simulink model "computed_torque_rl"  (R2021b)
settings: Solver=VariableStepAuto  StartTime=0  StopTime=3.6  RelTol=1e-3
values from neighbouring files (symbols this model uses):
  kd = 2*sqrt(kp)    [model_using.m]
  kp = 50700    [model_using.m]
  n = 100    [model_using.m]
libraries: slpidlib x4
settings Model: SimulationMode=accelerator  Creator=dell  LastModifiedBy=Admin
settings DataIOCC: SaveFormat=StructureWithTime
settings OptimizationCC: BlockReduction=off  BufferReuse=off
settings DebuggingCC: AlgebraicLoopMsg=none  UnconnectedInputMsg=none  UnconnectedOutputMsg=none  UnconnectedLineMsg=none
settings ExplorerConfigSet: SimMechanicsOpenEditorOnUpdate=off

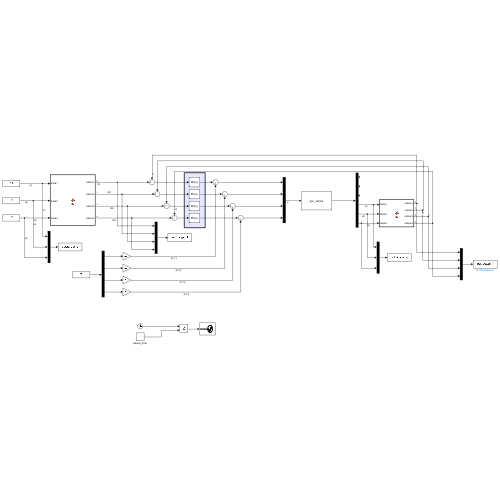
[thumbnail: Simulink's stored preview of the top-level diagram]
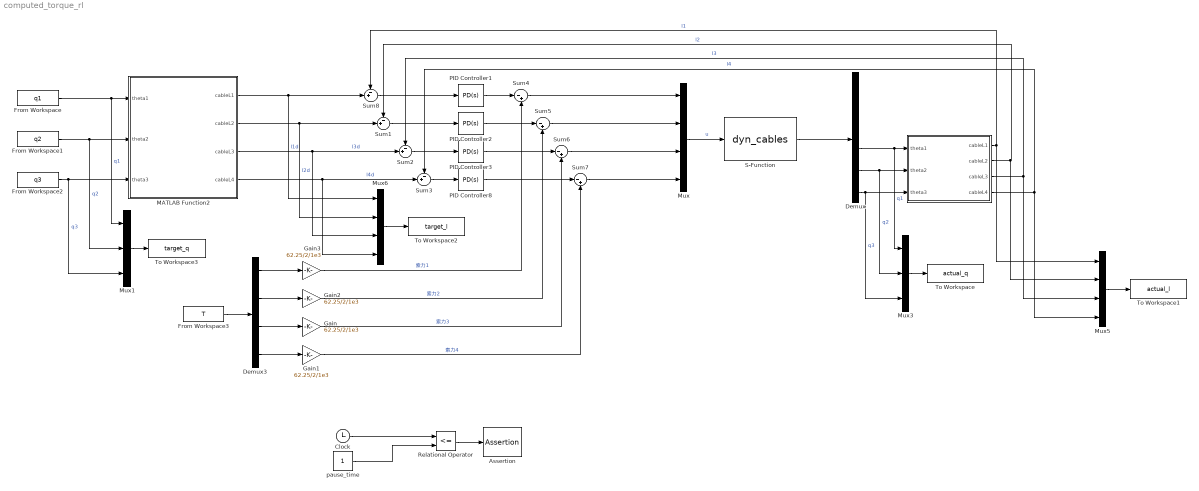
== system computed_torque_rl ==
  " " : MATLAB Function  TreatAsAtomicUnit=on
  Assertion : Assertion  AssertionFailFcn=set_param(bdroot,'SimulationCommand','pause'),disp(sprintf('\nSimulation paused.'))  StopWhenAssertionFail=off
  Clock : Clock
  Demux : Demux  Outputs=6
  Demux3 : Demux
  From Workspace : FromWorkspace  VariableName=q1
  From Workspace1 : FromWorkspace  VariableName=q2
  From Workspace2 : FromWorkspace  VariableName=q3
  From Workspace3 : FromWorkspace  VariableName=T
  Gain{,1..3} (4 alike) : Gain  Gain=62.25/2/1e3
  MATLAB Function2 : MATLAB Function  TreatAsAtomicUnit=on
  Mux : Mux
  Mux1 : Mux  Inputs=3
  Mux3 : Mux  Inputs=3
  Mux5 : Mux
  Mux6 : Mux
  PID Controller1 : slpidlib/PID Controller  Controller=PD  Form=Parallel  TimeDomain=Continuous-time  UseExternalTs=off  SampleTime=-1  IntegratorMethod=Forward Euler  FilterMethod=Forward Euler  ControllerParametersSource=internal  P=kp  I=-923.621241823871  D=kd  UseFilter=on  N=n  TunerSelectOption=Transfer Function Based (PID Tuner App)  InitialConditionSource=internal  InitialConditionForIntegrator=0  InitialConditionForFilter=0  DifferentiatorICPrevScaledInput=0  ExternalReset=none  TrackingMode=off  Kt=1  LimitOutput=off  SatLimitsSource=internal  UpperSaturationLimit=inf  LowerSaturationLimit=-inf  LinearizeAsGain=on  AntiWindupMode=none  Kb=1  POutMin=[]  POutMax=[]  IOutMin=[]  IOutMax=[]  DOutMin=[]  DOutMax=[]  NOutMin=[]  NOutMax=[]  SumOutMin=[]  SumOutMax=[]  SaturationOutMin=[]  SaturationOutMax=[]  PParamMin=[]  PParamMax=[]  IParamMin=[]  IParamMax=[]  DParamMin=[]  DParamMax=[]  NParamMin=[]  NParamMax=[]  KbParamMin=[]  KbParamMax=[]  KtParamMin=[]  KtParamMax=[]  KbOutMin=[]  KbOutMax=[]  KtOutMin=[]  KtOutMax=[]  IntegratorOutMin=[]  IntegratorOutMax=[]  FilterOutMin=[]  FilterOutMax=[]  SumI1OutMin=[]  SumI1OutMax=[]  SumI2OutMin=[]  SumI2OutMax=[]  SumI3OutMin=[]  SumI3OutMax=[]  SumI4OutMin=[]  SumI4OutMax=[]  SumDOutMin=[]  SumDOutMax=[]  DifferentiatorOutMin=[]  DifferentiatorOutMax=[]  FilterDiffOutCoefMin=[]  FilterDiffOutCoefMax=[]  ReciprocalOutMin=[]  ReciprocalOutMax=[]  SumDenOutMin=[]  SumDenOutMax=[]  SumNumOutMin=[]  SumNumOutMax=[]  DivideOutMin=[]  DivideOutMax=[]  UdiffTsProdOutMin=[]  UdiffTsProdOutMax=[]  NTsProdOutMin=[]  NTsProdOutMax=[]  UintegralTsProdOutMin=[]  UintegralTsProdOutMax=[]  UngainTsProdOutMin=[]  UngainTsProdOutMax=[]  IntegratorContinuousStateAttributes=''  IntegratorStateMustResolveToSignalObject=off  IntegratorRTWStateStorageClass=Auto  FilterContinuousStateAttributes=''  FilterStateMustResolveToSignalObject=off  FilterRTWStateStorageClass=Auto  ParallelPVariant=InternalParameters  IdealPVariant=Disabled  IVariant=Disabled  DVariant=InternalParameters  IntegratorVariant=Disabled  SatVariant=Disabled  AWVariant=Disabled  PCopyVariant=Disabled  TRVariant=Disabled  FdbkBlocksVariant=Forward  IdealPFdbkVariant=Disabled  SatFdbkVariant=Disabled  DerivativeFilterVariant=ContFilter  NVariant=InternalParameters  NCopyVariant=Disabled  FilterICVariant=InternalICsFilter  IntegratorICVariant=Disabled  ExternalResetVariant=Disabled  TRSumVariant=Passthrough  SumFdbkVariant=Disabled  SumVariant=Sum_PD  TsampFilterVariant=InternalTs  TsampNgainVariant=Passthrough  TsampIntegralVariant=Disabled_SignalSpec  ExternalSaturationOutDataTypeStr=Inherit: Same as second input
  PID Controller2 : slpidlib/PID Controller  Controller=PD  Form=Parallel  TimeDomain=Continuous-time  UseExternalTs=off  SampleTime=-1  IntegratorMethod=Forward Euler  FilterMethod=Forward Euler  ControllerParametersSource=internal  P=kp  I=-861163.925943885  D=kd  UseFilter=on  N=n  TunerSelectOption=Transfer Function Based (PID Tuner App)  InitialConditionSource=internal  InitialConditionForIntegrator=0  InitialConditionForFilter=0  DifferentiatorICPrevScaledInput=0  ExternalReset=none  TrackingMode=off  Kt=1  LimitOutput=off  SatLimitsSource=internal  UpperSaturationLimit=inf  LowerSaturationLimit=-inf  LinearizeAsGain=on  AntiWindupMode=none  Kb=1  POutMin=[]  POutMax=[]  IOutMin=[]  IOutMax=[]  DOutMin=[]  DOutMax=[]  NOutMin=[]  NOutMax=[]  SumOutMin=[]  SumOutMax=[]  SaturationOutMin=[]  SaturationOutMax=[]  PParamMin=[]  PParamMax=[]  IParamMin=[]  IParamMax=[]  DParamMin=[]  DParamMax=[]  NParamMin=[]  NParamMax=[]  KbParamMin=[]  KbParamMax=[]  KtParamMin=[]  KtParamMax=[]  KbOutMin=[]  KbOutMax=[]  KtOutMin=[]  KtOutMax=[]  IntegratorOutMin=[]  IntegratorOutMax=[]  FilterOutMin=[]  FilterOutMax=[]  SumI1OutMin=[]  SumI1OutMax=[]  SumI2OutMin=[]  SumI2OutMax=[]  SumI3OutMin=[]  SumI3OutMax=[]  SumI4OutMin=[]  SumI4OutMax=[]  SumDOutMin=[]  SumDOutMax=[]  DifferentiatorOutMin=[]  DifferentiatorOutMax=[]  FilterDiffOutCoefMin=[]  FilterDiffOutCoefMax=[]  ReciprocalOutMin=[]  ReciprocalOutMax=[]  SumDenOutMin=[]  SumDenOutMax=[]  SumNumOutMin=[]  SumNumOutMax=[]  DivideOutMin=[]  DivideOutMax=[]  UdiffTsProdOutMin=[]  UdiffTsProdOutMax=[]  NTsProdOutMin=[]  NTsProdOutMax=[]  UintegralTsProdOutMin=[]  UintegralTsProdOutMax=[]  UngainTsProdOutMin=[]  UngainTsProdOutMax=[]  IntegratorContinuousStateAttributes=''  IntegratorStateMustResolveToSignalObject=off  IntegratorRTWStateStorageClass=Auto  FilterContinuousStateAttributes=''  FilterStateMustResolveToSignalObject=off  FilterRTWStateStorageClass=Auto  ParallelPVariant=InternalParameters  IdealPVariant=Disabled  IVariant=Disabled  DVariant=InternalParameters  IntegratorVariant=Disabled  SatVariant=Disabled  AWVariant=Disabled  PCopyVariant=Disabled  TRVariant=Disabled  FdbkBlocksVariant=Forward  IdealPFdbkVariant=Disabled  SatFdbkVariant=Disabled  DerivativeFilterVariant=ContFilter  NVariant=InternalParameters  NCopyVariant=Disabled  FilterICVariant=InternalICsFilter  IntegratorICVariant=Disabled  ExternalResetVariant=Disabled  TRSumVariant=Passthrough  SumFdbkVariant=Disabled  SumVariant=Sum_PD  TsampFilterVariant=InternalTs  TsampNgainVariant=Passthrough  TsampIntegralVariant=Disabled_SignalSpec  ExternalSaturationOutDataTypeStr=Inherit: Same as second input
  PID Controller3 : slpidlib/PID Controller  Controller=PD  Form=Parallel  TimeDomain=Continuous-time  UseExternalTs=off  SampleTime=-1  IntegratorMethod=Forward Euler  FilterMethod=Forward Euler  ControllerParametersSource=internal  P=kp  I=-3010108.27344582  D=kd  UseFilter=on  N=n  TunerSelectOption=Transfer Function Based (PID Tuner App)  InitialConditionSource=internal  InitialConditionForIntegrator=0  InitialConditionForFilter=0  DifferentiatorICPrevScaledInput=0  ExternalReset=none  TrackingMode=off  Kt=1  LimitOutput=off  SatLimitsSource=internal  UpperSaturationLimit=inf  LowerSaturationLimit=-inf  LinearizeAsGain=on  AntiWindupMode=none  Kb=1  POutMin=[]  POutMax=[]  IOutMin=[]  IOutMax=[]  DOutMin=[]  DOutMax=[]  NOutMin=[]  NOutMax=[]  SumOutMin=[]  SumOutMax=[]  SaturationOutMin=[]  SaturationOutMax=[]  PParamMin=[]  PParamMax=[]  IParamMin=[]  IParamMax=[]  DParamMin=[]  DParamMax=[]  NParamMin=[]  NParamMax=[]  KbParamMin=[]  KbParamMax=[]  KtParamMin=[]  KtParamMax=[]  KbOutMin=[]  KbOutMax=[]  KtOutMin=[]  KtOutMax=[]  IntegratorOutMin=[]  IntegratorOutMax=[]  FilterOutMin=[]  FilterOutMax=[]  SumI1OutMin=[]  SumI1OutMax=[]  SumI2OutMin=[]  SumI2OutMax=[]  SumI3OutMin=[]  SumI3OutMax=[]  SumI4OutMin=[]  SumI4OutMax=[]  SumDOutMin=[]  SumDOutMax=[]  DifferentiatorOutMin=[]  DifferentiatorOutMax=[]  FilterDiffOutCoefMin=[]  FilterDiffOutCoefMax=[]  ReciprocalOutMin=[]  ReciprocalOutMax=[]  SumDenOutMin=[]  SumDenOutMax=[]  SumNumOutMin=[]  SumNumOutMax=[]  DivideOutMin=[]  DivideOutMax=[]  UdiffTsProdOutMin=[]  UdiffTsProdOutMax=[]  NTsProdOutMin=[]  NTsProdOutMax=[]  UintegralTsProdOutMin=[]  UintegralTsProdOutMax=[]  UngainTsProdOutMin=[]  UngainTsProdOutMax=[]  IntegratorContinuousStateAttributes=''  IntegratorStateMustResolveToSignalObject=off  IntegratorRTWStateStorageClass=Auto  FilterContinuousStateAttributes=''  FilterStateMustResolveToSignalObject=off  FilterRTWStateStorageClass=Auto  ParallelPVariant=InternalParameters  IdealPVariant=Disabled  IVariant=Disabled  DVariant=InternalParameters  IntegratorVariant=Disabled  SatVariant=Disabled  AWVariant=Disabled  PCopyVariant=Disabled  TRVariant=Disabled  FdbkBlocksVariant=Forward  IdealPFdbkVariant=Disabled  SatFdbkVariant=Disabled  DerivativeFilterVariant=ContFilter  NVariant=InternalParameters  NCopyVariant=Disabled  FilterICVariant=InternalICsFilter  IntegratorICVariant=Disabled  ExternalResetVariant=Disabled  TRSumVariant=Passthrough  SumFdbkVariant=Disabled  SumVariant=Sum_PD  TsampFilterVariant=InternalTs  TsampNgainVariant=Passthrough  TsampIntegralVariant=Disabled_SignalSpec  ExternalSaturationOutDataTypeStr=Inherit: Same as second input
  PID Controller8 : slpidlib/PID Controller  Controller=PD  Form=Parallel  TimeDomain=Continuous-time  UseExternalTs=off  SampleTime=-1  IntegratorMethod=Forward Euler  FilterMethod=Forward Euler  ControllerParametersSource=internal  P=kp  I=-2327391.8410066  D=kd  UseFilter=on  N=n  TunerSelectOption=Transfer Function Based (PID Tuner App)  InitialConditionSource=internal  InitialConditionForIntegrator=0  InitialConditionForFilter=0  DifferentiatorICPrevScaledInput=0  ExternalReset=none  TrackingMode=off  Kt=1  LimitOutput=off  SatLimitsSource=internal  UpperSaturationLimit=inf  LowerSaturationLimit=-inf  LinearizeAsGain=on  AntiWindupMode=none  Kb=1  POutMin=[]  POutMax=[]  IOutMin=[]  IOutMax=[]  DOutMin=[]  DOutMax=[]  NOutMin=[]  NOutMax=[]  SumOutMin=[]  SumOutMax=[]  SaturationOutMin=[]  SaturationOutMax=[]  PParamMin=[]  PParamMax=[]  IParamMin=[]  IParamMax=[]  DParamMin=[]  DParamMax=[]  NParamMin=[]  NParamMax=[]  KbParamMin=[]  KbParamMax=[]  KtParamMin=[]  KtParamMax=[]  KbOutMin=[]  KbOutMax=[]  KtOutMin=[]  KtOutMax=[]  IntegratorOutMin=[]  IntegratorOutMax=[]  FilterOutMin=[]  FilterOutMax=[]  SumI1OutMin=[]  SumI1OutMax=[]  SumI2OutMin=[]  SumI2OutMax=[]  SumI3OutMin=[]  SumI3OutMax=[]  SumI4OutMin=[]  SumI4OutMax=[]  SumDOutMin=[]  SumDOutMax=[]  DifferentiatorOutMin=[]  DifferentiatorOutMax=[]  FilterDiffOutCoefMin=[]  FilterDiffOutCoefMax=[]  ReciprocalOutMin=[]  ReciprocalOutMax=[]  SumDenOutMin=[]  SumDenOutMax=[]  SumNumOutMin=[]  SumNumOutMax=[]  DivideOutMin=[]  DivideOutMax=[]  UdiffTsProdOutMin=[]  UdiffTsProdOutMax=[]  NTsProdOutMin=[]  NTsProdOutMax=[]  UintegralTsProdOutMin=[]  UintegralTsProdOutMax=[]  UngainTsProdOutMin=[]  UngainTsProdOutMax=[]  IntegratorContinuousStateAttributes=''  IntegratorStateMustResolveToSignalObject=off  IntegratorRTWStateStorageClass=Auto  FilterContinuousStateAttributes=''  FilterStateMustResolveToSignalObject=off  FilterRTWStateStorageClass=Auto  ParallelPVariant=InternalParameters  IdealPVariant=Disabled  IVariant=Disabled  DVariant=InternalParameters  IntegratorVariant=Disabled  SatVariant=Disabled  AWVariant=Disabled  PCopyVariant=Disabled  TRVariant=Disabled  FdbkBlocksVariant=Forward  IdealPFdbkVariant=Disabled  SatFdbkVariant=Disabled  DerivativeFilterVariant=ContFilter  NVariant=InternalParameters  NCopyVariant=Disabled  FilterICVariant=InternalICsFilter  IntegratorICVariant=Disabled  ExternalResetVariant=Disabled  TRSumVariant=Passthrough  SumFdbkVariant=Disabled  SumVariant=Sum_PD  TsampFilterVariant=InternalTs  TsampNgainVariant=Passthrough  TsampIntegralVariant=Disabled_SignalSpec  ExternalSaturationOutDataTypeStr=Inherit: Same as second input
  Relational Operator : RelationalOperator  Operator=<=  OutDataTypeStr=boolean  RndMeth=Simplest
  S-Function : S-Function  FunctionName=dyn_cables  SFunctionDeploymentMode=off  EnableBusSupport=off
  Sum{1..3,8} (4 alike) : Sum  Inputs=-+|
  Sum{4..7} (4 alike) : Sum  Inputs=|-+
  To Workspace : ToWorkspace  VariableName=actual_q  SaveFormat=Timeseries  SampleTime=0.04
  To Workspace1 : ToWorkspace  VariableName=actual_l  SaveFormat=Timeseries  SampleTime=0.04
  To Workspace2 : ToWorkspace  VariableName=target_l  SaveFormat=Timeseries  SampleTime=0.04
  To Workspace3 : ToWorkspace  VariableName=target_q  SaveFormat=Timeseries  SampleTime=0.04
  pause_time : Constant
  wires:
  Mux/1 -> S-Function/1  "u"
  S-Function/1 -> Demux/1
  Sum4/1 -> Mux/1
  Sum8/1 -> PID Controller1/1
  MATLAB Function2/1(cableL1) -> Sum8/2, Mux6/1  "l1d"
  MATLAB Function2/2(cableL2) -> Sum1/2, Mux6/2  "l2d"
  Sum1/1 -> PID Controller2/1
  Sum5/1 -> Mux/2
  Sum6/1 -> Mux/3
  Sum2/1 -> PID Controller3/1
  MATLAB Function2/3(cableL3) -> Sum2/2, Mux6/3  "l3d"
  MATLAB Function2/4(cableL4) -> Sum3/2, Mux6/4  "l4d"
  Sum3/1 -> PID Controller8/1
  Sum7/1 -> Mux/4
  Demux/6 -> " "/3(theta3), Mux3/3  "q3"
  Demux/5 -> Mux3/2, " "/2(theta2)  "q2"
  Demux/4 -> Mux3/1, " "/1(theta1)  "q1"
  " "/4(cableL4) -> Sum3/1, Mux5/4  "l4"
  " "/3(cableL3) -> Mux5/3, Sum2/1  "l3"
  " "/2(cableL2) -> Mux5/2, Sum1/1  "l2"
  " "/1(cableL1) -> Sum8/1, Mux5/1  "l1"
  Gain1/1 -> Sum7/2  "索力4"
  Gain/1 -> Sum6/2  "索力3"
  Gain2/1 -> Sum5/2  "索力2"
  PID Controller2/1 -> Sum5/1
  PID Controller3/1 -> Sum6/1
  PID Controller8/1 -> Sum7/1
  Gain3/1 -> Sum4/2  "索力1"
  From Workspace3/1 -> Demux3/1
  Demux3/4 -> Gain1/1
  Demux3/3 -> Gain/1
  Demux3/2 -> Gain2/1
  Demux3/1 -> Gain3/1
  Mux3/1 -> To Workspace/1
  Mux5/1 -> To Workspace1/1
  Mux6/1 -> To Workspace2/1
  PID Controller1/1 -> Sum4/1
  From Workspace2/1 -> Mux1/3, MATLAB Function2/3(theta3)  "q3"
  From Workspace1/1 -> MATLAB Function2/2(theta2), Mux1/2  "q2"
  From Workspace/1 -> Mux1/1, MATLAB Function2/1(theta1)  "q1"
  Mux1/1 -> To Workspace3/1
  Clock/1 -> Relational Operator/1
  pause_time/1 -> Relational Operator/2
  Relational Operator/1 -> Assertion/1

== matlab function computed_torque_rl/  ==
  data: cableL1 output; cableL2 output; cableL3 output; cableL4 output; theta1 input; theta2 input; theta3 input
function [cableL1,cableL2,cableL3,cableL4]  = IK(theta1,theta2,theta3)
        JacobianNumber = zeros(3,4);cableL1=0;cableL2=0;cableL3=0;cableL4=0;
        %% 机器人下肢参数
        Lt = 0.465;   % 单位mm
        Lc = 0.369;   % 单位mm
        D0 = 1.0585;    % 单位m
        pi = 3.14159;
        R = 0.008;
        
        %% 牵引点tow point（简写为TP）相关参数输入。
        % 注：样机系统中这8个参数由Nokov系统每次试验先采集后处理获得后方进行控制试验。
        Dcap1 = 0.3985;       % 大腿牵索点（牵索点1）与髋关节中心沿大腿轴线的距离。
        TP1ToT = 0.084;      %索1的牵索点（即牵索点1）到大腿连杆的垂线距离，即大腿袖带半径Rtc。
        
        Dcap2 = 0.208;        % 小腿牵索点（牵索点2）与膝关节中心沿小腿轴线的距离。
        TP2ToC = 0.059;     %索2的牵索点（即牵索点2）到小腿连杆的垂线距离，即小腿袖带半径Rcc。

        Dcap3 = 0.0885;   % 足部牵索点（牵索点3）与踝关节中心沿足部轴线的距
%         TP3ToF = -0.050;      % 足部袖带1半径，即牵索点（牵索点3）垂直于足部轴线的距离。
        TP3ToF = -0.100;      % 为避免干涉，改为-0.1

        Dcap4 = 0.1335;   % 足部牵索点（牵索点4）与踝关节中心沿足部轴线的距
        TP4ToF = 0.059;       % 足部袖带2半径，即牵索点（牵索点4）垂直于足部轴线的距离。
        
        %% 出索点SCAP（Spool cable attachment point：绕线轮与绳索连接点，即出索点）坐标输入。
        % 出索点坐标。注：优化过程中出索点X轴坐标是不变的。
        xP1 = 0.875;
        yP1 = 0.952;   
        SCAP1 = [xP1;yP1];   %M1电机（出索点1）的X、Y轴坐标
        
        xP2 = -0.875;
        yP2 = 0.940;
        SCAP2 = [xP2;yP2];  
        
        xP3 = -0.875;
        yP3 = 1.610;
        SCAP3 = [xP3;yP3];  
        
        xP4 = 0.875;
        yP4 = 1.200;
        SCAP4 = [xP4;yP4]; 
        
    %% 牵引点tow point坐标（TowPointLocation）计算。Homogeneous Transformation Matrix：齐次变换矩阵
     % HTM_TPi：牵引点i在机器人基坐标系中的齐次变换矩阵。
    %  Location_TowPoint：牵引点i在机器人基坐标系中的坐标，符号为Ri。

    %     HTM_TP1 = transl(0,D0,0)*trotx(pi)*trotz(-pi/2)*trotz(theta1)*transl(Dcap1,TP1ToT,0);  %将髋关节牵索点（牵索点1）从局部坐标变换到全局坐标的齐次变换矩阵
    %     Location_TowPoint1=HTM_TP1(1:2,4);  % r = Matrix(1:3,2:4)：表示取Matrix的1~3行中的2~4列构成新的矩阵，即牵索点1在基坐标系中的坐标。
        xa1 = Dcap1*sin(theta1) + TP1ToT*cos(theta1); 
        ya1 = D0 + Dcap1*cos(theta1) - TP1ToT*sin(theta1); 
        Location_TowPoint1 = [xa1;ya1];     % 牵引点1坐标计算

    %     HTM_TP2 = transl(0,D0,0)*trotx(pi)*trotz(-pi/2)*trotz(theta1)*transl(Lt,0,0)*trotz(theta2)*transl(Dcap2,-TP2ToC,0);
    %     Location_TowPoint2 = HTM_TP2(1:2,4);  %牵索点2在基坐标系中的坐标。
        xa2 = Lt*sin(theta1) + Dcap2*sin(theta1 + theta2) - TP2ToC*cos(theta1 + theta2); 
        ya2 = D0 + Lt*cos(theta1) + Dcap2*cos(theta1 + theta2) + TP2ToC*sin(theta1 + theta2); 
        Location_TowPoint2 = [xa2;ya2];     % 牵引点2坐标计算

    %     HTM_TP3 = transl(0,D0,0)*trotx(pi)*trotz(-pi/2)*trotz(theta1)*transl(Lt,0,0)*trotz(theta2)*transl(Lc,0,0)*trotz(pi/2)*trotz(theta3)*transl(Dcap3,-TP3ToF,0);
    %     Location_TowPoint3 = HTM_TP3(1:2,4);   %牵索点3在基坐标系中的坐标。
    % Location_TowPoint3已修正
        xa3 = Lt*sin(theta1) + Lc*sin(theta1 + theta2) + Dcap3*cos(theta1 + theta2 + theta3) - TP3ToF*sin(theta1 + theta2 + theta3); 
        ya3 = D0 + Lt*cos(theta1) + Lc*cos(theta1 + theta2) - Dcap3*sin(theta1 + theta2 + theta3) - TP3ToF*cos(theta1 + theta2 + theta3); 
        Location_TowPoint3 = [xa3;ya3];     % 牵引点3坐标计算

    %     HTM_TP4 = transl(0,D0,0)*trotx(pi)*trotz(-pi/2)*trotz(theta1)*transl(Lt,0,0)*trotz(theta2)*transl(Lc,0,0)*trotz(pi/2)*trotz(theta3)*transl(Dcap4,TP4ToF,0);
    %     Location_TowPoint4 = HTM_TP4(1:2,4);  %牵索点4在基坐标系中的坐标。
        xa4 = Lt*sin(theta1) + Lc*sin(theta1 + theta2) + Dcap4*cos(theta1 + theta2 + theta3) - TP4ToF*sin(theta1 + theta2 + theta3); 
        ya4 = D0 + Lt*cos(theta1) + Lc*cos(theta1 + theta2) - Dcap4*sin(theta1 + theta2 + theta3) - TP4ToF*cos(theta1 + theta2 + theta3); 
        Location_TowPoint4 = [xa4;ya4];     % 牵引点4坐标计算
        
        %%
         beta1 = acos(R/norm(Location_TowPoint1 - SCAP1))-atan(norm(yP1-ya1)/norm(xP1-xa1));
         beta2 = acos(R/norm(Location_TowPoint2 - SCAP2))-atan(norm(yP2-ya2)/norm(xP2-xa2));
         beta3 = acos(R/norm(Location_TowPoint3 - SCAP3))-atan(norm(yP3-ya3)/norm(xP3-xa3));
         beta4 = acos(R/norm(Location_TowPoint4 - SCAP4))-atan(norm(yP4-ya4)/norm(xP4-xa4));
%          beta4 = acos(real(complex(R/norm(Location_TowPoint4 - SCAP4))))-atan(norm(yP4-ya4)/norm(xP4-xa4));
         %实际出索点
         outpoint1 = [xP1-R*cos(beta1);yP1-R*sin(beta1)];
         outpoint2 = [xP2+R*cos(beta2);yP2-R*sin(beta2)];
         outpoint3 = [xP3+R*cos(beta3);yP3-R*sin(beta3)];
         outpoint4 = [xP4-R*cos(beta4);yP4-R*sin(beta4)];
         
         %绳长
%          cableL1 = 0.939296033169760-norm(Location_TowPoint1 - outpoint1);
%          cableL2 = 1.116051436394486-norm(Location_TowPoint2 - outpoint2);
%          cableL3 = 0.998100002957835-norm(Location_TowPoint3 - outpoint3);
%          cableL4 = 0.985007754695478-norm(Location_TowPoint4 - outpoint4);

         cableL1 = norm(Location_TowPoint1 - outpoint1);
         cableL2 = norm(Location_TowPoint2 - outpoint2);
         cableL3 = norm(Location_TowPoint3 - outpoint3);
         cableL4 = norm(Location_TowPoint4 - outpoint4);

        % 计算绳索的单位矢量 CableLocationVector：绳索在基坐标系中的向量，简写为CableLV。
     % Cable Location Unit Vector：绳索在基坐标系中的单位向量，简写为CLUnitVector。
%         CableLV1 = outpoint1 - Location_TowPoint1;  % 索1（连接电机1与牵索点1的索）在基坐标系中的向量
%         UnitVector1 = CableLV1/sqrt(CableLV1(1)^2+CableLV1(2)^2);  % 索1在基坐标系中的单位向量，或说索1拉力的单位方向向量。
% 
%         CableLV2 = outpoint2 - Location_TowPoint2;  % 索2（连接电机2与牵索点2的索）在基坐标系中的向量
%         UnitVector2=CableLV2/sqrt(CableLV2(1)^2+CableLV2(2)^2);  % 索2在基坐标系中的单位向量
% 
%         CableLV3 = outpoint3 - Location_TowPoint3;  % 索3（连接电机3与牵索点3的索）在基坐标系中的向量
%         UnitVector3=CableLV3/sqrt(CableLV3(1)^2+CableLV3(2)^2);  % 索3在基坐标系中的单位向量
% 
%         CableLV4 = outpoint4 - Location_TowPoint4;  % 索4（连接电机4与牵索点4的索）在基坐标系中的向量
%         UnitVector4=CableLV4/sqrt(CableLV4(1)^2+CableLV4(2)^2);  % 索4在基坐标系中的单位向
% 
%          % %求解力的雅克比矩阵JT（论文中写为JL）。
%     DeltaR1theta1 = [Dcap1*cos(theta1) - TP1ToT*sin(theta1);
%                      -Dcap1*sin(theta1) - TP1ToT*cos(theta1)];
%     DeltaR1theta2 = [0;0];
%     DeltaR1theta3 = [0;0];
% 
%     DeltaR2theta1= [Lt*cos(theta1) + Dcap2*cos(theta1 + theta2) + TP2ToC*sin(theta1 + theta2);
%                     -Lt*sin(theta1) - Dcap2*sin(theta1 + theta2) + TP2ToC*cos(theta1 + theta2)];
%     DeltaR2theta2= [Dcap2*cos(theta1 + theta2) + TP2ToC*sin(theta1 + theta2);
%                     - Dcap2*sin(theta1 + theta2) + TP2ToC*cos(theta1 + theta2)];
%     DeltaR2theta3 = [0;0];
% 
%     % 已修改。并校对无误
%     DeltaR3theta1= [Lt*cos(theta1) + Lc*cos(theta1 + theta2) - Dcap3*sin(theta1 + theta2 + theta3) - TP3ToF*cos(theta1 + theta2 + theta3); 
%                     -Lt*sin(theta1) - Lc*sin(theta1 + theta2) - Dcap3*cos(theta1 + theta2 + theta3) + TP3ToF*sin(theta1 + theta2 + theta3)];
%     DeltaR3theta2= [Lc*cos(theta1 + theta2) - Dcap3*sin(theta1 + theta2 + theta3) - TP3ToF*cos(theta1 + theta2 + theta3); 
%                     - Lc*sin(theta1 + theta2) - Dcap3*cos(theta1 + theta2 + theta3) + TP3ToF*sin(theta1 + theta2 + theta3)];
%     DeltaR3theta3= [- Dcap3*sin(theta1 + theta2 + theta3) - TP3ToF*cos(theta1 + theta2 + theta3); 
%                     - Dcap3*cos(theta1 + theta2 + theta3) + TP3ToF*sin(theta1 + theta2 + theta3)];
%     
%     DeltaR4theta1= [Lt*cos(theta1) + Lc*cos(theta1 + theta2) - Dcap4*sin(theta1 + theta2 + theta3) - TP4ToF*cos(theta1 + theta2 + theta3)
%                     - Lt*sin(theta1) - Lc*sin(theta1 + theta2) - Dcap4*cos(theta1 + theta2 + theta3) + TP4ToF*sin(theta1 + theta2 + theta3)];
%     DeltaR4theta2= [Lc*cos(theta1 + theta2) - Dcap4*sin(theta1 + theta2 + theta3) - TP4ToF*cos(theta1 + theta2 + theta3)
%                     - Lc*sin(theta1 + theta2) - Dcap4*cos(theta1 + theta2 + theta3) + TP4ToF*sin(theta1 + theta2 + theta3)];
%     DeltaR4theta3= [- Dcap4*sin(theta1 + theta2 + theta3) - TP4ToF*cos(theta1 + theta2 + theta3)
%                     - Dcap4*cos(theta1 + theta2 + theta3) + TP4ToF*sin(theta1 + theta2 + theta3)];
% 
% 
%    
%     JacobianNumber = [UnitVector1'*DeltaR1theta1  UnitVector2'*DeltaR2theta1  UnitVector3'*DeltaR3theta1  UnitVector4'*DeltaR4theta1;
%                       UnitVector1'*DeltaR1theta2  UnitVector2'*DeltaR2theta2  UnitVector3'*DeltaR3theta2  UnitVector4'*DeltaR4theta2;
%                       UnitVector1'*DeltaR1theta3  UnitVector2'*DeltaR2theta3  UnitVector3'*DeltaR3theta3  UnitVector4'*DeltaR4theta3];  % 力的雅克比矩阵JL（表达式形式），是速度雅克比矩阵的转置。

%       % 求解索力的通解。两种方法求解结果相同
%       coder.extrinsic('Motion_To_NullspaceAndCLength');
%       NullSpace = Motion_To_NullspaceAndCLength(JacobianNumber);
  
end

== matlab function computed_torque_rl/MATLAB Function2 ==
  data: cableL1 output; cableL2 output; cableL3 output; cableL4 output; theta1 input; theta2 input; theta3 input
function [cableL1,cableL2,cableL3,cableL4]  = IK(theta1,theta2,theta3)
        JacobianNumber = zeros(3,4);cableL1=0;cableL2=0;cableL3=0;cableL4=0;
        %% 机器人下肢参数
        Lt = 0.465;   % 单位mm
        Lc = 0.369;   % 单位mm
        D0 = 1.0585;    % 单位m
        pi = 3.14159;
        R = 0.008;
        
        %% 牵引点tow point（简写为TP）相关参数输入。
        % 注：样机系统中这8个参数由Nokov系统每次试验先采集后处理获得后方进行控制试验。
        Dcap1 = 0.3985;       % 大腿牵索点（牵索点1）与髋关节中心沿大腿轴线的距离。
        TP1ToT = 0.084;      %索1的牵索点（即牵索点1）到大腿连杆的垂线距离，即大腿袖带半径Rtc。
        
        Dcap2 = 0.208;        % 小腿牵索点（牵索点2）与膝关节中心沿小腿轴线的距离。
        TP2ToC = 0.059;     %索2的牵索点（即牵索点2）到小腿连杆的垂线距离，即小腿袖带半径Rcc。

        Dcap3 = 0.0885;   % 足部牵索点（牵索点3）与踝关节中心沿足部轴线的距
%         TP3ToF = -0.050;      % 足部袖带1半径，即牵索点（牵索点3）垂直于足部轴线的距离。
        TP3ToF = -0.100;      % 为避免干涉，改为-0.1

        Dcap4 = 0.1335;   % 足部牵索点（牵索点4）与踝关节中心沿足部轴线的距
        TP4ToF = 0.059;       % 足部袖带2半径，即牵索点（牵索点4）垂直于足部轴线的距离。
        
        %% 出索点SCAP（Spool cable attachment point：绕线轮与绳索连接点，即出索点）坐标输入。
        % 出索点坐标。注：优化过程中出索点X轴坐标是不变的。
        xP1 = 0.875;
        yP1 = 0.952;   
        SCAP1 = [xP1;yP1];   %M1电机（出索点1）的X、Y轴坐标
        
        xP2 = -0.875;
        yP2 = 0.940;
        SCAP2 = [xP2;yP2];  
        
        xP3 = -0.875;
        yP3 = 1.610;
        SCAP3 = [xP3;yP3];  
        
        xP4 = 0.875;
        yP4 = 1.200;
        SCAP4 = [xP4;yP4]; 
        
    %% 牵引点tow point坐标（TowPointLocation）计算。Homogeneous Transformation Matrix：齐次变换矩阵
     % HTM_TPi：牵引点i在机器人基坐标系中的齐次变换矩阵。
    %  Location_TowPoint：牵引点i在机器人基坐标系中的坐标，符号为Ri。

    %     HTM_TP1 = transl(0,D0,0)*trotx(pi)*trotz(-pi/2)*trotz(theta1)*transl(Dcap1,TP1ToT,0);  %将髋关节牵索点（牵索点1）从局部坐标变换到全局坐标的齐次变换矩阵
    %     Location_TowPoint1=HTM_TP1(1:2,4);  % r = Matrix(1:3,2:4)：表示取Matrix的1~3行中的2~4列构成新的矩阵，即牵索点1在基坐标系中的坐标。
        xa1 = Dcap1*sin(theta1) + TP1ToT*cos(theta1); 
        ya1 = D0 + Dcap1*cos(theta1) - TP1ToT*sin(theta1); 
        Location_TowPoint1 = [xa1;ya1];     % 牵引点1坐标计算

    %     HTM_TP2 = transl(0,D0,0)*trotx(pi)*trotz(-pi/2)*trotz(theta1)*transl(Lt,0,0)*trotz(theta2)*transl(Dcap2,-TP2ToC,0);
    %     Location_TowPoint2 = HTM_TP2(1:2,4);  %牵索点2在基坐标系中的坐标。
        xa2 = Lt*sin(theta1) + Dcap2*sin(theta1 + theta2) - TP2ToC*cos(theta1 + theta2); 
        ya2 = D0 + Lt*cos(theta1) + Dcap2*cos(theta1 + theta2) + TP2ToC*sin(theta1 + theta2); 
        Location_TowPoint2 = [xa2;ya2];     % 牵引点2坐标计算

    %     HTM_TP3 = transl(0,D0,0)*trotx(pi)*trotz(-pi/2)*trotz(theta1)*transl(Lt,0,0)*trotz(theta2)*transl(Lc,0,0)*trotz(pi/2)*trotz(theta3)*transl(Dcap3,-TP3ToF,0);
    %     Location_TowPoint3 = HTM_TP3(1:2,4);   %牵索点3在基坐标系中的坐标。
    % Location_TowPoint3已修正
        xa3 = Lt*sin(theta1) + Lc*sin(theta1 + theta2) + Dcap3*cos(theta1 + theta2 + theta3) - TP3ToF*sin(theta1 + theta2 + theta3); 
        ya3 = D0 + Lt*cos(theta1) + Lc*cos(theta1 + theta2) - Dcap3*sin(theta1 + theta2 + theta3) - TP3ToF*cos(theta1 + theta2 + theta3); 
        Location_TowPoint3 = [xa3;ya3];     % 牵引点3坐标计算

    %     HTM_TP4 = transl(0,D0,0)*trotx(pi)*trotz(-pi/2)*trotz(theta1)*transl(Lt,0,0)*trotz(theta2)*transl(Lc,0,0)*trotz(pi/2)*trotz(theta3)*transl(Dcap4,TP4ToF,0);
    %     Location_TowPoint4 = HTM_TP4(1:2,4);  %牵索点4在基坐标系中的坐标。
        xa4 = Lt*sin(theta1) + Lc*sin(theta1 + theta2) + Dcap4*cos(theta1 + theta2 + theta3) - TP4ToF*sin(theta1 + theta2 + theta3); 
        ya4 = D0 + Lt*cos(theta1) + Lc*cos(theta1 + theta2) - Dcap4*sin(theta1 + theta2 + theta3) - TP4ToF*cos(theta1 + theta2 + theta3); 
        Location_TowPoint4 = [xa4;ya4];     % 牵引点4坐标计算
        
        %%
         beta1 = acos(R/norm(Location_TowPoint1 - SCAP1))-atan(norm(yP1-ya1)/norm(xP1-xa1));
         beta2 = acos(R/norm(Location_TowPoint2 - SCAP2))-atan(norm(yP2-ya2)/norm(xP2-xa2));
         beta3 = acos(R/norm(Location_TowPoint3 - SCAP3))-atan(norm(yP3-ya3)/norm(xP3-xa3));
         beta4 = acos(R/norm(Location_TowPoint4 - SCAP4))-atan(norm(yP4-ya4)/norm(xP4-xa4));
         %实际出索点
         outpoint1 = [xP1-R*cos(beta1);yP1-R*sin(beta1)];
         outpoint2 = [xP2+R*cos(beta2);yP2-R*sin(beta2)];
         outpoint3 = [xP3+R*cos(beta3);yP3-R*sin(beta3)];
         outpoint4 = [xP4-R*cos(beta4);yP4-R*sin(beta4)];
         
         %绳长
%          cableL1 = 0.939296033169760-norm(Location_TowPoint1 - outpoint1);
%          cableL2 = 1.116051436394486-norm(Location_TowPoint2 - outpoint2);
%          cableL3 = 0.998100002957835-norm(Location_TowPoint3 - outpoint3);
%          cableL4 = 0.985007754695478-norm(Location_TowPoint4 - outpoint4);

         cableL1 = norm(Location_TowPoint1 - outpoint1);
         cableL2 = norm(Location_TowPoint2 - outpoint2);
         cableL3 = norm(Location_TowPoint3 - outpoint3);
         cableL4 = norm(Location_TowPoint4 - outpoint4);

        % 计算绳索的单位矢量 CableLocationVector：绳索在基坐标系中的向量，简写为CableLV。
     % Cable Location Unit Vector：绳索在基坐标系中的单位向量，简写为CLUnitVector。
%         CableLV1 = outpoint1 - Location_TowPoint1;  % 索1（连接电机1与牵索点1的索）在基坐标系中的向量
%         UnitVector1 = CableLV1/sqrt(CableLV1(1)^2+CableLV1(2)^2);  % 索1在基坐标系中的单位向量，或说索1拉力的单位方向向量。
% 
%         CableLV2 = outpoint2 - Location_TowPoint2;  % 索2（连接电机2与牵索点2的索）在基坐标系中的向量
%         UnitVector2=CableLV2/sqrt(CableLV2(1)^2+CableLV2(2)^2);  % 索2在基坐标系中的单位向量
% 
%         CableLV3 = outpoint3 - Location_TowPoint3;  % 索3（连接电机3与牵索点3的索）在基坐标系中的向量
%         UnitVector3=CableLV3/sqrt(CableLV3(1)^2+CableLV3(2)^2);  % 索3在基坐标系中的单位向量
% 
%         CableLV4 = outpoint4 - Location_TowPoint4;  % 索4（连接电机4与牵索点4的索）在基坐标系中的向量
%         UnitVector4=CableLV4/sqrt(CableLV4(1)^2+CableLV4(2)^2);  % 索4在基坐标系中的单位向
% 
%          % %求解力的雅克比矩阵JT（论文中写为JL）。
%     DeltaR1theta1 = [Dcap1*cos(theta1) - TP1ToT*sin(theta1);
%                      -Dcap1*sin(theta1) - TP1ToT*cos(theta1)];
%     DeltaR1theta2 = [0;0];
%     DeltaR1theta3 = [0;0];
% 
%     DeltaR2theta1= [Lt*cos(theta1) + Dcap2*cos(theta1 + theta2) + TP2ToC*sin(theta1 + theta2);
%                     -Lt*sin(theta1) - Dcap2*sin(theta1 + theta2) + TP2ToC*cos(theta1 + theta2)];
%     DeltaR2theta2= [Dcap2*cos(theta1 + theta2) + TP2ToC*sin(theta1 + theta2);
%                     - Dcap2*sin(theta1 + theta2) + TP2ToC*cos(theta1 + theta2)];
%     DeltaR2theta3 = [0;0];
% 
%     % 已修改。并校对无误
%     DeltaR3theta1= [Lt*cos(theta1) + Lc*cos(theta1 + theta2) - Dcap3*sin(theta1 + theta2 + theta3) - TP3ToF*cos(theta1 + theta2 + theta3); 
%                     -Lt*sin(theta1) - Lc*sin(theta1 + theta2) - Dcap3*cos(theta1 + theta2 + theta3) + TP3ToF*sin(theta1 + theta2 + theta3)];
%     DeltaR3theta2= [Lc*cos(theta1 + theta2) - Dcap3*sin(theta1 + theta2 + theta3) - TP3ToF*cos(theta1 + theta2 + theta3); 
%                     - Lc*sin(theta1 + theta2) - Dcap3*cos(theta1 + theta2 + theta3) + TP3ToF*sin(theta1 + theta2 + theta3)];
%     DeltaR3theta3= [- Dcap3*sin(theta1 + theta2 + theta3) - TP3ToF*cos(theta1 + theta2 + theta3); 
%                     - Dcap3*cos(theta1 + theta2 + theta3) + TP3ToF*sin(theta1 + theta2 + theta3)];
%     
%     DeltaR4theta1= [Lt*cos(theta1) + Lc*cos(theta1 + theta2) - Dcap4*sin(theta1 + theta2 + theta3) - TP4ToF*cos(theta1 + theta2 + theta3)
%                     - Lt*sin(theta1) - Lc*sin(theta1 + theta2) - Dcap4*cos(theta1 + theta2 + theta3) + TP4ToF*sin(theta1 + theta2 + theta3)];
%     DeltaR4theta2= [Lc*cos(theta1 + theta2) - Dcap4*sin(theta1 + theta2 + theta3) - TP4ToF*cos(theta1 + theta2 + theta3)
%                     - Lc*sin(theta1 + theta2) - Dcap4*cos(theta1 + theta2 + theta3) + TP4ToF*sin(theta1 + theta2 + theta3)];
%     DeltaR4theta3= [- Dcap4*sin(theta1 + theta2 + theta3) - TP4ToF*cos(theta1 + theta2 + theta3)
%                     - Dcap4*cos(theta1 + theta2 + theta3) + TP4ToF*sin(theta1 + theta2 + theta3)];
% 
% 
%    
%     JacobianNumber = [UnitVector1'*DeltaR1theta1  UnitVector2'*DeltaR2theta1  UnitVector3'*DeltaR3theta1  UnitVector4'*DeltaR4theta1;
%                       UnitVector1'*DeltaR1theta2  UnitVector2'*DeltaR2theta2  UnitVector3'*DeltaR3theta2  UnitVector4'*DeltaR4theta2;
%                       UnitVector1'*DeltaR1theta3  UnitVector2'*DeltaR2theta3  UnitVector3'*DeltaR3theta3  UnitVector4'*DeltaR4theta3];  % 力的雅克比矩阵JL（表达式形式），是速度雅克比矩阵的转置。

%       % 求解索力的通解。两种方法求解结果相同
%       coder.extrinsic('Motion_To_NullspaceAndCLength');
%       NullSpace = Motion_To_NullspaceAndCLength(JacobianNumber);
  
end
